simulink model "test_noncircular"  (R2017b)
settings: Solver=VariableStepAuto  StartTime=0.0  StopTime=inf  RelTol=1e-3
undefined symbols (not defined in the file or in its folder): F
libraries: dspspect3 x1, zc706fmc234_lib x1
settings Model: SimulationMode=accelerator  Creator=ppradhan  LastModifiedBy=ppradhan
settings CodeAppCC: StateflowObjectComments=on

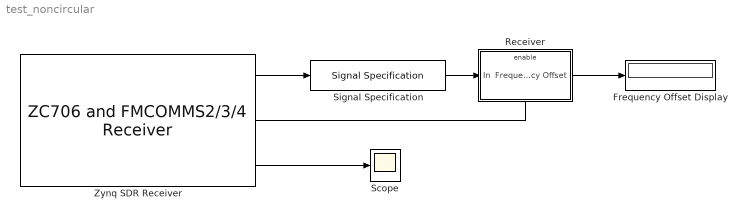
== system test_noncircular ==
  Frequency Offset Display : Display
  Receiver : Subsystem
      mask Display: disp('Receiver')
  Scope : Scope
  Signal Specification : SignalSpecification  SampleTime=4096/1e6
  Zynq SDR Receiver : zc706fmc234_lib/ZC706 and  FMCOMMS2//3//4  Receiver  IPAddress=192.168.3.2  CenterFrequencySource=Dialog  CenterFrequency=5e9  GainSource=AGC Slow Attack  Gain=1  ChannelMapping=1  BasebandSampleRate=1000000  EnableBurstMode=off  NumFramesInBurst=20  OutputDataType=double  SamplesPerFrame=4096  LostSamplesOutputPort=on  RSSIOutputPort=off  DMATimeoutValue=1  blockMode=Normal  SimulateUsing=Code generation  EnableQuadratureTracking=on  EnableRFDCTracking=on  EnableBasebandDCTracking=on  BypassUserLogic=on  ShowAdvancedProperties=on  ShowInternalProperties=off  subDeviceList=zynqReceiver  sdrExecutionMode=HW  dataUDPPort=-1  ctrlUDPPort=-1  SourceSelect=RF data  SourceConfiguration1=1023  FIRCoefficientSize=[128;64]  FIRCoefficients=[190 -88 329 -40 239 -99 -24 -349 -377 -611 -573 -604 -395 -229 66 239 394 350 227 -46 -300 -534 -593 -506 -221 137 512 737 765 526 103 -420 -852 -1069 -947 -512 156 841 1341 1450 1100 333 -638 -1531 -2028 -1922 -1152 115 1544 2677 3099 2535 997 -1205 -3479 -5095 -5345 -3750 -199 4965 11002 16895 21580 24172 24172 21580 16895 11002 4965 -199 -3750 -5345 -5095 -3479 -1205 997 2535 3099 2677 1544 115 -1152 -1922 -2028 -1531 -638 333 1100 1450 1341 841 156 -512 -947 -1069 -852 -420 103 526 765 737 512 137 -221 -506 -593 -534 -300 -46 227 350 394 239 66 -229 -395 -604 -573 -611 -377 -349 -24 -99 239 -40 329 -88 190;-2 -86 -41 -219 -201 -366 -356 -417 -302 -170 122 431 801 1074 1229 1125 756 78 -814 -1813 -2698 -3256 -3236 -2467 -837 1620 4756 8277 11816 14953 17302 18558 18558 17302 14953 11816 8277 4756 1620 -837 -2467 -3236 -3256 -2698 -1813 -814 78 756 1125 1229 1074 801 431 122 -170 -302 -417 -356 -366 -201 -219 -41 -86 -2 0 0 0 0 0 0 0 0 0 0 0 0 0 0 0 0 0 0 0 0 0 0 0 0 0 0 0 0 0 0 0 0 0 0 0 0 0 0 0 0 0 0 0 0 0 0 0 0 0 0 0 0 0 0 0 0 0 0 0 0 0 0 0 0]  FIRGain=[-12;-12]  FIRDecimInterpFactor=[4;4]  AnalogFilterCutoff=[831851;831851]  FilterPathRates=[1024000000 32000000 16000000 8000000 4000000 1000000;1024000000 32000000 16000000 8000000 4000000 1000000]  FilterDesignTypeForTx=CustomFilterFromOther  FilterDesignTypeForRx=CustomFilter  BISTLoopbackConfig=No Loopback  BISTPRBSMode=PRBS Disable  BISTToneMode=Tone Disable  BISTToneFrequency=F/32  BISTToneLevel=-6  BISTChannelMask=0  DataIsComplex=on
      settings: SourceProductName=Communications System Toolbox Support Package for Xilinx Zynq-Based Radio  SourceProductBaseCode=XILINXZYNQ
  wires:
  Zynq SDR Receiver/2 -> Receiver/Enable
  Receiver/1(Frequency Offset) -> Frequency Offset Display/1
  Zynq SDR Receiver/3 -> Scope/1
  Zynq SDR Receiver/1 -> Signal Specification/1
  Signal Specification/1 -> Receiver/1(In)

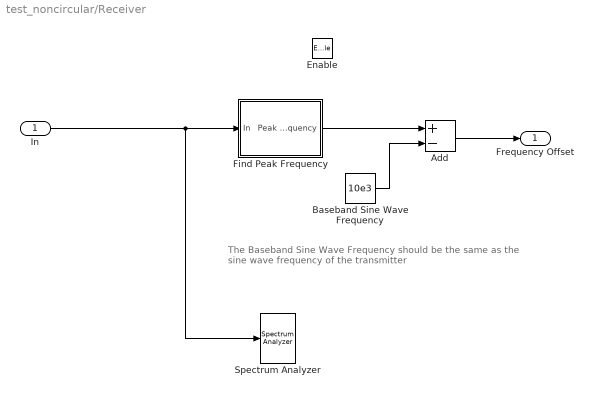
== system test_noncircular/Receiver ==
  note: The Baseband Sine Wave Frequency should be the same as
      | the sine wave frequency of the transmitter
  In : Inport
  Enable : EnablePort
  Add : Sum  Inputs=+-
  Baseband Sine Wave Frequency : Constant  Value=10e3
  Find Peak Frequency : Subsystem
      mask Display: disp('Find Peak\nFrequency')
  Spectrum Analyzer : SpectrumAnalyzer
  Frequency Offset : Outport
  wires:
  In/1 -> Find Peak Frequency/1(In), Spectrum Analyzer/1
  Find Peak Frequency/1(Peak Frequency) -> Add/1
  Baseband Sine Wave Frequency/1 -> Add/2
  Add/1 -> Frequency Offset/1

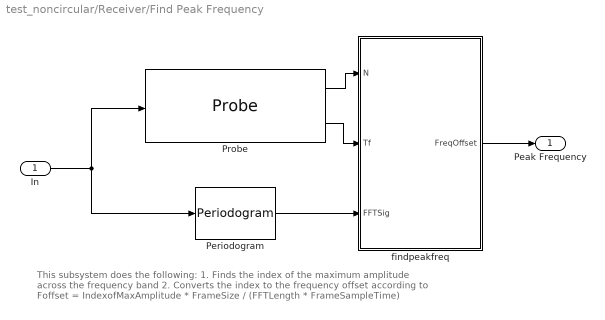
== system test_noncircular/Receiver/Find Peak Frequency ==
  note: This subsystem does the following:
      | 1.  Finds the index of the maximum amplitude across the frequency band
      | 2.  Converts the index to the frequency offset according to
      | Foffset = IndexofMaxAmplitude * FrameSize / (FFTLength * FrameSampleTime)
  In : Inport
  Periodogram : dspspect3/Periodogram  measurement=Power spectral density  wintype=Hamming  Rs=50  beta=5  winsamp=Symmetric  FFTImplementation=Auto  inheritFFT=off  fftsize=4096  navg=2  inheritTs=on  Ts=1
      settings: SourceProductName=DSP System Toolbox  SourceProductBaseCode=DS
  Probe : Probe  ProbeComplexSignal=off
  findpeakfreq : MATLAB Function  TreatAsAtomicUnit=on
  Peak Frequency : Outport
  wires:
  Periodogram/1 -> findpeakfreq/3(FFTSig)
  Probe/1 -> findpeakfreq/1(N)
  Probe/2 -> findpeakfreq/2(Tf)
  findpeakfreq/1(FreqOffset) -> Peak Frequency/1
  In/1 -> Periodogram/1, Probe/1

== matlab function test_noncircular/Receiver/Find Peak Frequency/findpeakfreq ==
  data: N input; FreqOffset output; Tf input; FFTSig input
function FreqOffset  = findpeakfreq(N, Tf, FFTSig)
% Find peak frequency
% N - frame size
% Tf - frame sample time
% FFTSig - result of FFT

%#codegen

FFTSize = length(FFTSig);
FFTSig = fftshift(FFTSig);
[~, maxIdx] = max(FFTSig); % Find index of max magnitude
OffsetIdx = maxIdx-1-FFTSize/2; % Convert to index symmetric with 0
Ts = Tf(1)/N; % Sample time
delta_f = 1/Ts/FFTSize; % Frequency resolution of FFT
FreqOffset = OffsetIdx*delta_f;% Map offset index back to frequency
